simulink library "csu_mmp_mems_messsage_processing_lib"  (R2014b)
settings: Solver=ode45  StartTime=0.0  StopTime=10.0  RelTol=1e-3
undefined symbols (not defined in the file): mnm_accel_range, mnm_gyro_range, spc_mem1_accel_bias, spc_mem1_rate_bias, spc_mem2_accel_bias, spc_mem2_rate_bias, spc_mem3_accel_bias, spc_mem3_rate_bias
libraries: simulink x1, util_info_lib x1
settings Model: Creator=escrane  LastModifiedBy=mstewart

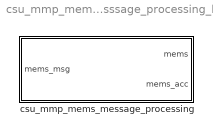
== system csu_mmp_mems_messsage_processing_lib ==
  csu_mmp_mems_message_processing : Subsystem

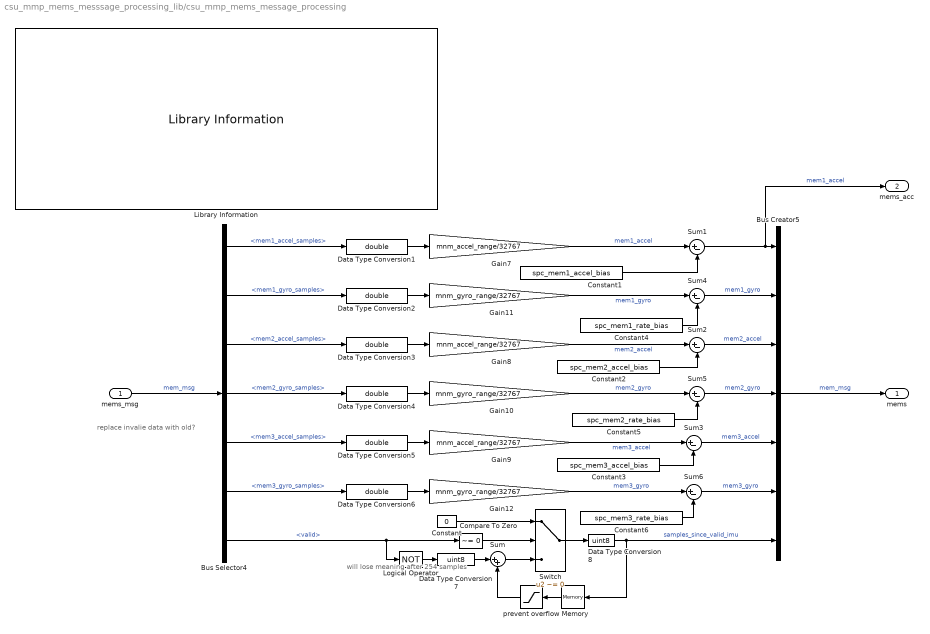
== system csu_mmp_mems_messsage_processing_lib/csu_mmp_mems_message_processing ==
  note: will lose meaning after 254 samples
  note: replace invalie data with old?
  mems_msg : Inport
  Bus Creator5 : BusCreator  Inputs=7
  Bus Selector4 : BusSelector  OutputSignals=mem1_accel_samples,mem1_gyro_samples,mem2_accel_samples,mem2_gyro_samples,mem3_accel_samples,mem3_gyro_samples,valid
  Compare To Zero : simulink/Logic and Bit Operations/Compare To Zero  relop=~=  OutDataTypeStr=boolean
  Constant : Constant  Value=0  OutDataTypeStr=uint8
  Constant1 : Constant  Value=spc_mem1_accel_bias  OutDataTypeStr=double
  Constant2 : Constant  Value=spc_mem2_accel_bias  OutDataTypeStr=double
  Constant3 : Constant  Value=spc_mem3_accel_bias  OutDataTypeStr=double
  Constant4 : Constant  Value=spc_mem1_rate_bias  OutDataTypeStr=double
  Constant5 : Constant  Value=spc_mem2_rate_bias  OutDataTypeStr=double
  Constant6 : Constant  Value=spc_mem3_rate_bias  OutDataTypeStr=double
  Data Type Conversion{1..6} (6 alike) : DataTypeConversion  OutDataTypeStr=double
  Data Type Conversion7 : DataTypeConversion  OutDataTypeStr=uint8
  Data Type Conversion8 : DataTypeConversion  OutDataTypeStr=uint8
  Gain10 : Gain  Gain=mnm_gyro_range/32767  OutDataTypeStr=double
  Gain11 : Gain  Gain=mnm_gyro_range/32767  OutDataTypeStr=double
  Gain12 : Gain  Gain=mnm_gyro_range/32767  OutDataTypeStr=double
  Gain7 : Gain  Gain=mnm_accel_range/32767  OutDataTypeStr=double
  Gain8 : Gain  Gain=mnm_accel_range/32767  OutDataTypeStr=double
  Gain9 : Gain  Gain=mnm_accel_range/32767  OutDataTypeStr=double
  Library Information : util_info_lib/Library Information  owner='escrane'
  Logical Operator : Logic  Operator=NOT  AllPortsSameDT=off  OutDataTypeStr=boolean
  Memory : Memory  X0=uint8(0)  InheritSampleTime=on
  Sum : Sum  Inputs=|++
  Sum{1..6} (6 alike) : Sum  Inputs=|+-
  Switch : Switch  Criteria=u2 ~= 0
  prevent overflow : Saturate  UpperLimit=254  LowerLimit=0
  mems : Outport
  mems_acc : Outport  Port=2
  wires:
  Constant1/1 -> Sum1/2
  Constant6/1 -> Sum6/2
  Gain12/1 -> Sum6/1  "mem3_gyro"
  Constant5/1 -> Sum5/2
  Constant4/1 -> Sum4/2
  Gain11/1 -> Sum4/1  "mem1_gyro"
  Gain10/1 -> Sum5/1  "mem2_gyro"
  Gain9/1 -> Sum3/1  "mem3_accel"
  Gain8/1 -> Sum2/1  "mem2_accel"
  Constant3/1 -> Sum3/2
  Constant2/1 -> Sum2/2
  Gain7/1 -> Sum1/1  "mem1_accel"
  Data Type Conversion8/1 -> Bus Creator5/7, Memory/1  "samples_since_valid_imu"
  Switch/1 -> Data Type Conversion8/1
  prevent overflow/1 -> Sum/2
  Logical Operator/1 -> Data Type Conversion7/1
  Data Type Conversion7/1 -> Sum/1
  Compare To Zero/1 -> Switch/2
  Sum/1 -> Switch/3
  Constant/1 -> Switch/1
  Memory/1 -> prevent overflow/1
  Bus Selector4/7 -> Compare To Zero/1, Logical Operator/1  "<valid>"
  Sum3/1 -> Bus Creator5/5  "mem3_accel"
  Sum6/1 -> Bus Creator5/6  "mem3_gyro"
  Sum5/1 -> Bus Creator5/4  "mem2_gyro"
  Sum2/1 -> Bus Creator5/3  "mem2_accel"
  Sum4/1 -> Bus Creator5/2  "mem1_gyro"
  Sum1/1 -> mems_acc/1, Bus Creator5/1  "mem1_accel"
  Data Type Conversion6/1 -> Gain12/1
  Data Type Conversion5/1 -> Gain9/1
  Data Type Conversion4/1 -> Gain10/1
  Data Type Conversion3/1 -> Gain8/1
  Data Type Conversion2/1 -> Gain11/1
  Data Type Conversion1/1 -> Gain7/1
  Bus Selector4/6 -> Data Type Conversion6/1  "<mem3_gyro_samples>"
  Bus Selector4/5 -> Data Type Conversion5/1  "<mem3_accel_samples>"
  Bus Selector4/4 -> Data Type Conversion4/1  "<mem2_gyro_samples>"
  Bus Selector4/3 -> Data Type Conversion3/1  "<mem2_accel_samples>"
  Bus Selector4/2 -> Data Type Conversion2/1  "<mem1_gyro_samples>"
  Bus Selector4/1 -> Data Type Conversion1/1  "<mem1_accel_samples>"
  mems_msg/1 -> Bus Selector4/1  "mem_msg"
  Bus Creator5/1 -> mems/1  "mem_msg"
